simulink model "Filter_Refrenced_model"  (R2020b)
settings: Solver=VariableStepAuto  StartTime=0.0  StopTime=10.0  MaxStep=0.001  RelTol=1e-3
settings Model: Creator=HP  LastModifiedBy=HP
settings DataIOCC: SaveOutput=off  SaveTime=off

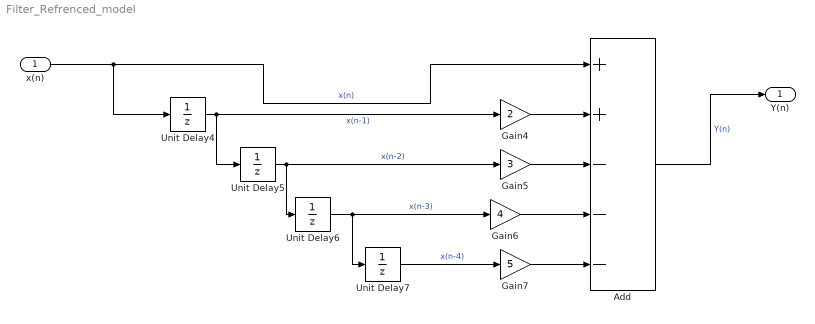
== system Filter_Refrenced_model ==
  x(n) : Inport  OutDataTypeStr=double  PortDimensions=1  SampleTime=0
  Add : Sum  Inputs=++---
  Gain4 : Gain  Gain=2
  Gain5 : Gain  Gain=3
  Gain6 : Gain  Gain=4
  Gain7 : Gain  Gain=5
  Unit Delay{4..7} (4 alike) : UnitDelay  SampleTime=-1  HasFrameUpgradeWarning=on
  Y(n) : Outport  OutDataTypeStr=double  PortDimensions=1  SampleTime=0
  wires:
  Gain7/1 -> Add/5
  Unit Delay4/1 -> Unit Delay5/1, Gain4/1  "x(n-1)"
  Gain6/1 -> Add/4
  Unit Delay5/1 -> Unit Delay6/1, Gain5/1  "x(n-2)"
  x(n)/1 -> Add/1, Unit Delay4/1  "x(n)"
  Unit Delay6/1 -> Unit Delay7/1, Gain6/1  "x(n-3)"
  Unit Delay7/1 -> Gain7/1  "x(n-4)"
  Gain4/1 -> Add/2
  Gain5/1 -> Add/3
  Add/1 -> Y(n)/1  "Y(n)"
